simulink model "Get_RE_Signal"  (R2013a)
settings: Solver=FixedStepDiscrete  StartTime=0.0  StopTime=60  RelTol=1e-3
undefined symbols (not defined in the file): ts
libraries: arduino_io_lib x4
settings Model: Creator=cell  LastModifiedBy=cell
settings OptimizationCC: OptimizeModelRefInitCode=on  LifeSpan=1
settings DebuggingCC: StrictBusMsg=Warning
settings HardwareCC: ProdBitPerInt=16  ProdBitPerPointer=8  ProdIntDivRoundTo=Zero  ProdEndianess=LittleEndian  ProdWordSize=8  ProdHWDeviceType=Atmel->AVR
settings RTWCC: SystemTargetFile=realtime.tlc  GenerateMakefile=off  TemplateMakefile=realtime.tmf  Description=Run on Target Hardware  RTWVerbose=off  ProcessScript=realtime_make_rtw_hook
settings CodeAppCC: IgnoreCustomStorageClasses=off
settings STFCustomTargetCC: TargetLibSuffix=.a  GenerateSampleERTMain=on  CombineOutputUpdateFcns=on  ERTCustomFileBanners=on  SupportContinuousTime=off  SupportNonInlinedSFcns=off  MATLABClassNameForMDSCustomization=Simulink.SoftwareTarget.ERTCustomization  SystemTargetFile=realtime.tlc
settings ERTTargetCC: ParMdlRefBuildCompliant=off  CompOptLevelCompliant=off  ConcurrentExecutionCompliant=off  ERTFirstTimeCompliant=off  ModelStepFunctionPrototypeControlCompliant=off  CPPClassGenCompliant=off  ERTCustomFileTemplate=realtime_file_process.tlc

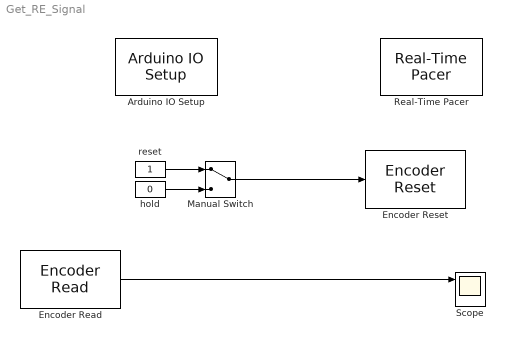
== system Get_RE_Signal ==
  Arduino IO Setup : arduino_io_lib/Arduino IO Setup  Priority=3  arduinoVar=Existing workspace arduino variable #1  workspaceVarName=a  comPort=DEMO
  Encoder Read : arduino_io_lib/Encoder Read  arduinoVar=Existing workspace arduino variable #1  encNum=1  pinA=2  pinB=3  DbDl=0  T=ts
  Encoder Reset : arduino_io_lib/Encoder Reset  arduinoVar=Existing workspace arduino variable #1  encNum=1  T=ts
  Manual Switch : ManualSwitch
  Real-Time Pacer : arduino_io_lib/Real-Time Pacer  simTimePerRealTime=1
  Scope : Scope  NumInputPorts=3
      settings: TimeRange=10  YMin=-1000~-1~-1  YMax=1000~1~1
  hold : Constant  Value=0
  reset : Constant
  wires:
  reset/1 -> Manual Switch/1
  hold/1 -> Manual Switch/2
  Manual Switch/1 -> Encoder Reset/1
  Encoder Read/1 -> Scope/1
